simulink model "struttura_hinf"  (R2015b)
settings: Solver=VariableStepAuto  StartTime=0.0  StopTime=10.0  RelTol=1e-3
values from neighbouring files (symbols this model uses):
  den1 = [10000 1]    [h_infinito.m]    (also in mu_controller.m)
  den2 = [0.001 1]    [h_infinito.m]    (also in mu_controller.m = [0.01 1])
  dend = 1    [h_infinito.m]    (also in mu_controller.m)
  gain1 = 72    [h_infinito.m]    (also in mu_controller.m = 80)
  gain2 = 0.01    [h_infinito.m]    (also in mu_controller.m = 0.002)
  gaind = 0.1    [h_infinito.m]    (also in mu_controller.m)
  Greal = sysic    [model_building.m]
  num1 = [1 1]    [h_infinito.m]    (also in mu_controller.m = [0.1 1])
  num2 = [10 1]    [h_infinito.m]    (also in mu_controller.m = [100 1])
  numd = 1    [h_infinito.m]    (also in mu_controller.m)
undefined symbols (not defined in the file or in its folder): Ks_inf
settings Model: Creator=michele  LastModifiedBy=michele

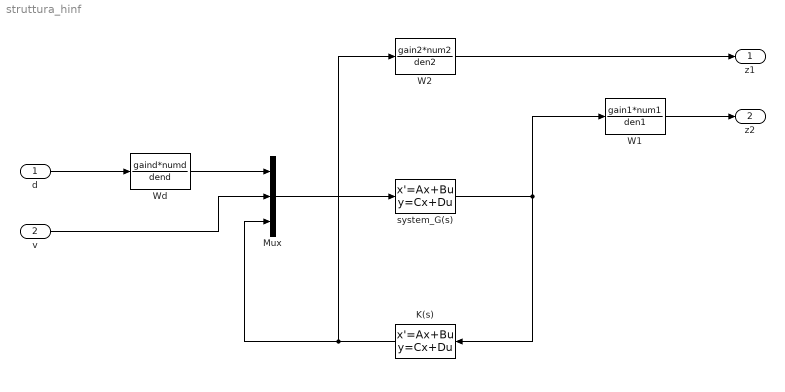
== system struttura_hinf ==
  d : Inport
  v : Inport  Port=2
  K(s) : StateSpace  A=Ks_inf.a  B=Ks_inf.b  C=Ks_inf.c  D=Ks_inf.d  X0=0
  Mux : Mux  Inputs=3
  W1 : TransferFcn  Numerator=gain1*num1  Denominator=den1
  W2 : TransferFcn  Numerator=gain2*num2  Denominator=den2
  Wd : TransferFcn  Numerator=gaind*numd  Denominator=dend
  system_G(s) : StateSpace  A=Greal.NominalValue.a  B=Greal.NominalValue.b  C=Greal.NominalValue.c  D=Greal.NominalValue.d  X0=0
  z1 : Outport
  z2 : Outport  Port=2
  wires:
  system_G(s)/1 -> K(s)/1, W1/1
  Mux/1 -> system_G(s)/1
  K(s)/1 -> W2/1, Mux/3
  Wd/1 -> Mux/1
  d/1 -> Wd/1
  v/1 -> Mux/2
  W2/1 -> z1/1
  W1/1 -> z2/1
